simulink model "SILsim"  (R2024a)
settings: Solver=ode8  StartTime=0.0  StopTime=inf  FixedStep=SampleTime  RelTol=1e-3
values from neighbouring files (symbols this model uses):
  Arm = [ ... (first row only)    [launch.m]
  CDDrone = 0.01    [launch.m]
  CDval = 0.008    [launch.m]
  g = 9.81    [launch.m]
  m = 1    [launch.m]
  m_to_mm = 1000    [launch.m]
  prop_inertia = (1/12) * 0.015 * 0.127^2    (= 2.016125e-05)    [launch.m]
  R = 0.127    [launch.m]
  ref_height = 76    [launch.m]
  ref_lat = 437818446e-7    (= 43.7818446)    [launch.m]
  ref_lon = -794679715e-7    (= -79.4679715)    [launch.m]
  rotorRPMMax = 10000    [launch.m]
  rotorTimeConst = 0.05    [launch.m]
  SampleTime = 0.004    [launch.m]
  tilt_speed = [0; pi/4; 0]    [launch.m]
undefined symbols (not defined in the file or in its folder): contact, control, ddx, ddy, ddz, dx, dy, dz, fractalcoef, lastVh, p, pitch, q, r, roll, X, Y, yaw, Z
libraries: sharedutil x3, robotcorelib x2, simulink x2, shared6dof x1, simulink_extras x1, matrix_library x1, aerolibatmos2 x1, sensorgpslib x1, mspsensorlib x1, aerolibanimutils x1, uavutilslib x1
(part 2 of 2)

== system SILsim/Quad Tiltrotor Dynamics/Airframe/Motor Forces and Torques/If transitioning/Multirotor Subsystem/Rotor Subsystem/Force Calculation ==
  Coeff. Thrust : Inport
  Omega : Inport  Port=2
  rho : Inport  Port=3
  Tilt angle : Inport  Port=4
  Arm : Inport  Port=5
  Components : Subsystem
  Fx Sign : Subsystem
  Induced Vel Calc : Subsystem
  Math Function3 : Math  Operator=square  SignedPower=on
  Mux : Mux  Inputs=3
  Product6 : Product  Inputs=3
  R3 : Gain  Gain=R*R*pi*R*R
  Induced Velocity : Outport
  Thrust : Outport  Port=2
  wires:
  Coeff. Thrust/1 -> Product6/1
  Math Function3/1 -> R3/1
  Induced Vel Calc/1(Vh) -> Induced Velocity/1
  R3/1 -> Product6/2
  rho/1 -> Product6/3
  Omega/1 -> Math Function3/1
  Product6/1 -> Components/3(F), Induced Vel Calc/1(Thrust)  "F"
  Arm/1 -> Fx Sign/1(Arm)
  Mux/1 -> Thrust/1
  Fx Sign/1(Xsign) -> Components/1(Sign)
  Tilt angle/1 -> Components/2(Tilt angle)
  Components/1(Fx) -> Mux/1
  Components/2(Fy) -> Mux/2
  Components/3(Fz) -> Mux/3

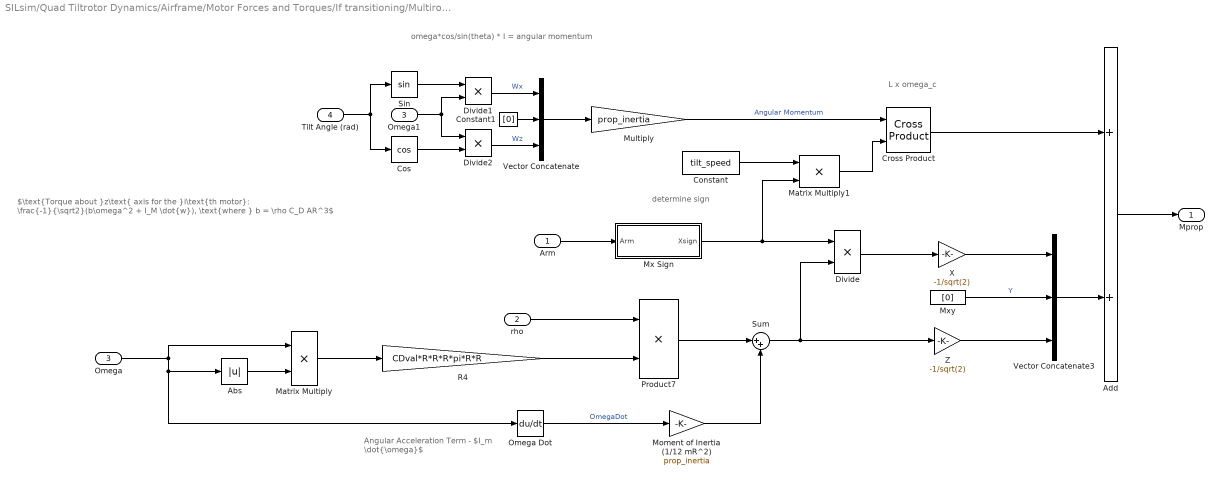
== system SILsim/Quad Tiltrotor Dynamics/Airframe/Motor Forces and Torques/If transitioning/Multirotor Subsystem/Rotor Subsystem/Moment Calculation ==
  note: determine sign
  note: L x omega_c
  note: omega*cos/sin(theta) * I = angular momentum
  note: $\text{Torque about }z\text{ axis for the }i\text{th motor}: \frac{-1}{\sqrt2}(b\omega^2 + I_M \dot{w}), \text{where } b = \rho C_D AR^3$
  note: Angular Acceleration Term - $I_m \dot{\omega}$
  Arm : Inport
  rho : Inport  Port=2
  Omega : Inport  Port=3
  Tilt Angle (rad) : Inport  Port=4
  Abs : Abs  SaturateOnIntegerOverflow=off
  Add : Sum
  Constant : Constant  Value=tilt_speed
  Constant1 : Constant  Value=[0]
  Cos : Trigonometry  Operator=cos
  Cross Product : matrix_library/Cross Product
  Divide : Product  Inputs=**
  Divide1 : Product  Inputs=**
  Divide2 : Product  Inputs=**
  Matrix Multiply : Product
  Matrix Multiply1 : Product
  Moment of Inertia (1/12 mR^2) : Gain  Gain=prop_inertia
  Multiply : Gain  Gain=prop_inertia
  Mx Sign : Subsystem
  Mxy : Constant  Value=[0]
  Omega Dot : Derivative
  Omega1 : InportShadow  Port=3
  Product7 : Product
  R4 : Gain  Gain=CDval*R*R*R*pi*R*R
  Sin : Trigonometry
  Sum : Sum  Inputs=|++
  Vector Concatenate : Concatenate  NumInputs=3
  Vector Concatenate3 : Concatenate  NumInputs=3
  X : Gain  Gain=-1/sqrt(2)
  Z : Gain  Gain=-1/sqrt(2)
  Mprop : Outport
  wires:
  R4/1 -> Product7/2
  rho/1 -> Product7/1
  Omega/1 -> Omega Dot/1, Abs/1, Matrix Multiply/1
  Omega Dot/1 -> Moment of Inertia (1/12 mR^2)/1  "OmegaDot"
  Sum/1 -> Z/1, Divide/2
  Product7/1 -> Sum/1
  Moment of Inertia (1/12 mR^2)/1 -> Sum/2
  Z/1 -> Vector Concatenate3/3
  Divide/1 -> X/1
  Mxy/1 -> Vector Concatenate3/2  "Y"
  Arm/1 -> Mx Sign/1(Arm)
  Mx Sign/1(Xsign) -> Divide/1, Matrix Multiply1/2
  Matrix Multiply/1 -> R4/1
  Abs/1 -> Matrix Multiply/2
  Tilt Angle (rad)/1 -> Cos/1, Sin/1
  Cos/1 -> Divide2/2
  Sin/1 -> Divide1/1
  Divide1/1 -> Vector Concatenate/1  "Wx"
  Vector Concatenate/1 -> Multiply/1
  Multiply/1 -> Cross Product/1  "Angular Momentum"
  Cross Product/1 -> Add/1
  Divide2/1 -> Vector Concatenate/3  "Wz"
  Constant1/1 -> Vector Concatenate/2
  Omega1/1 -> Divide2/1, Divide1/2
  Matrix Multiply1/1 -> Cross Product/2
  Constant/1 -> Matrix Multiply1/1
  X/1 -> Vector Concatenate3/1
  Vector Concatenate3/1 -> Add/2
  Add/1 -> Mprop/1

== system SILsim/Quad Tiltrotor Dynamics/Airframe/Motor Forces and Torques/If transitioning/Multirotor Subsystem/Rotor Subsystem/Tilted Ct Estimator ==
  note: - calculate ct/c0 from both estimators
      | - use tilt angle to perform a weighted average
  note: Accurate method:
      |
      | - model the tilt in ansys and find the thrust variation
  note: Possible simplified method:
      |
      | - stick to vrs dynamics from non tilted state for transitioning part -> more conservative
      | - do some interpolation between tilted and non tilted estimators
  Vz : Inport
  rpm : Inport  Port=2
  tilt_angle : Inport  Port=3
  Abs : Abs  SaturateOnIntegerOverflow=off
  Calculate Ct : Product  Inputs=**
  Ct/C0 State Switcher : Subsystem
  Ct0 estimator for RPM : Polyval  Coefs=[0.000000000012185, -0.000000274732884, 0.008305365728125]
  Divide1 : Product  Inputs=*/
  Tilt Normalization : Subsystem
  Vh Calculator : Polyval  Coefs=[-5.17622414362771e-09, 0.000822973507549008, 0.0232660553338375]
  Weighted Average Ct/C0 Fit : Subsystem
  Ct : Outport
  wires:
  Vh Calculator/1 -> Divide1/2  "Vh"
  Ct/C0 State Switcher/1(Out1) -> Calculate Ct/1  "Ct/C0"
  Divide1/1 -> Ct/C0 State Switcher/1(" Vz/Vh"), Weighted Average Ct/C0 Fit/1(Vz/Vh)  "Vz/Vh"
  rpm/1 -> Abs/1
  Abs/1 -> Vh Calculator/1, Ct0 estimator for RPM/1
  Ct0 estimator for RPM/1 -> Calculate Ct/2  "Ct0"
  Vz/1 -> Divide1/1
  Calculate Ct/1 -> Ct/1  "Ct"
  Weighted Average Ct/C0 Fit/1(Ct/Ct0) -> Ct/C0 State Switcher/2(Ct/C0 Fit)
  tilt_angle/1 -> Tilt Normalization/1(Angle)
  Tilt Normalization/1(%) -> Weighted Average Ct/C0 Fit/2(tilt %)
  Weighted Average Ct/C0 Fit/2(Ct/Ct0 Past Fit) -> Ct/C0 State Switcher/3(Ct/Ct0 Past Fit)

== system SILsim/Quad Tiltrotor Dynamics/Airframe/Motor Forces and Torques/If Tilted/Multirotor Subsystem/Rotor Subsystem/Ct Estimator/Ct//C0 State Switcher ==
  " Vz/Vh" : Inport
  Ct/C0 Fit : Inport  Port=2
  " Vz/Vh1" : InportShadow
  Constant : Constant  Value=1.00463796511
  If : If  IfExpression=u1 >= -2.828427125 & u1 <= 0  ElseIfExpressions=u1 < -2.828427125
  If Action Subsystem : Subsystem  TreatAsAtomicUnit=on
  If Action Subsystem1 : Subsystem  TreatAsAtomicUnit=on
  If Action Subsystem2 : Subsystem  TreatAsAtomicUnit=on
  Merge : Merge  Inputs=3
  Scope1 : Scope
  Out1 : Outport
  wires:
  If Action Subsystem2/1(Out1) -> Merge/3
  If/3 -> If Action Subsystem2/Action  "climb"
  If/1 -> If Action Subsystem/Action  "descent"
  If Action Subsystem/1(Out1) -> Merge/1
  " Vz/Vh"/1 -> If/1
  If/2 -> If Action Subsystem1/Action  "past curve fit"
  Merge/1 -> Scope1/1, Out1/1
  Ct/C0 Fit/1 -> If Action Subsystem/1(In1)
  Constant/1 -> If Action Subsystem2/1("  ")
  If Action Subsystem1/1(" ") -> Merge/2
  " Vz/Vh1"/1 -> If Action Subsystem1/1(" Vz/Vh")

== system SILsim/Quad Tiltrotor Dynamics/Airframe/Motor Forces and Torques/If Tilted/Multirotor Subsystem/Rotor Subsystem/Force Calculation/Fx Sign ==
  Arm : Inport
  Sign : Signum
  X selector : Selector  InputPortWidth=3  IndexOptions=Index vector (dialog)  Indices=[1]  OutputSizes=1
  Xsign : Outport
  wires:
  Arm/1 -> X selector/1
  X selector/1 -> Sign/1
  Sign/1 -> Xsign/1

== system SILsim/Quad Tiltrotor Dynamics/Airframe/Motor Forces and Torques/If Tilted/Multirotor Subsystem/Rotor Subsystem/Force Calculation/Induced Vel Calc ==
  Thrust : Inport
  Denom : Constant  Value=2*1.225*pi*R^2
  Divide : Product  Inputs=*/
  Sqrt : Sqrt  OutDataTypeStr=double
  Vh : Outport
  wires:
  Denom/1 -> Divide/2
  Divide/1 -> Sqrt/1
  Sqrt/1 -> Vh/1
  Thrust/1 -> Divide/1

== system SILsim/Quad Tiltrotor Dynamics/Airframe/Motor Forces and Torques/If Tilted/Multirotor Subsystem/Rotor Subsystem/Moment Calculation/Mx Sign ==
  Arm : Inport
  Sign : Signum
  X selector : Selector  InputPortWidth=3  IndexOptions=Index vector (dialog)  Indices=[1]  OutputSizes=1
  Xsign : Outport
  wires:
  Arm/1 -> X selector/1
  X selector/1 -> Sign/1
  Sign/1 -> Xsign/1

== system SILsim/Quad Tiltrotor Dynamics/Airframe/Motor Forces and Torques/If non tilted/Multirotor Subsystem/Rotor Subsystem/Force Calculation/Induced Vel Calc ==
  Thrust : Inport
  Denom : Constant  Value=2*1.225*pi*R^2
  Divide : Product  Inputs=*/
  Saturation : Saturate  UpperLimit=inf  LowerLimit=0
  Sqrt : Sqrt  OutDataTypeStr=double
  Vh : Outport
  wires:
  Denom/1 -> Divide/2
  Divide/1 -> Saturation/1
  Sqrt/1 -> Vh/1
  Thrust/1 -> Divide/1
  Saturation/1 -> Sqrt/1

== system SILsim/Quad Tiltrotor Dynamics/Airframe/Motor Forces and Torques/If non tilted/Multirotor Subsystem/Rotor Subsystem/Non Tilted Ct estimator/Ct//C0 State Switcher ==
  note: add random number variations to VRS thrust to simulate thrust fluctuations
  " Vz/Vh" : Inport
  Ct/C0 Fit : Inport  Port=2
  " Vz/Vh1" : InportShadow
  Climb : Subsystem  TreatAsAtomicUnit=on
  Constant : Constant  Value=0.9905
  Descent : Subsystem  TreatAsAtomicUnit=on
  If : If  IfExpression=u1 >= -2 & u1 <= 0  ElseIfExpressions=u1 < -2
  Merge : Merge  Inputs=3
  Past Curve Fit : Subsystem  TreatAsAtomicUnit=on
  Ct/Ct0 : Outport
  wires:
  Past Curve Fit/1(" ") -> Merge/2
  Climb/1(Out1) -> Merge/3
  If/3 -> Climb/Action
  If/1 -> Descent/Action
  If/2 -> Past Curve Fit/Action
  Ct/C0 Fit/1 -> Descent/1(Ct_Ct0)
  " Vz/Vh1"/1 -> Past Curve Fit/1(" Vz/Vh")
  Constant/1 -> Climb/1("  ")
  Merge/1 -> Ct/Ct0/1
  " Vz/Vh"/1 -> If/1
  Descent/1(Outport) -> Merge/1

== system SILsim/Quad Tiltrotor Dynamics/Airframe/Motor Forces and Torques/If transitioning/Multirotor Subsystem/Rotor Subsystem/Force Calculation/Components ==
  Sign : Inport
  Tilt angle : Inport  Port=2
  F : Inport  Port=3
  Constant : Constant  Value=0
  Cos : Trigonometry
  Divide : Product  Inputs=**
  Matrix Multiply : Product
  Matrix Multiply1 : Product
  Sin : Trigonometry  Operator=cos
  Fx : Outport
  Fy : Outport  Port=2
  Fz : Outport  Port=3
  wires:
  Tilt angle/1 -> Cos/1, Sin/1
  Sign/1 -> Divide/1
  Sin/1 -> Matrix Multiply1/1
  Constant/1 -> Fy/1  "Fy"
  Cos/1 -> Matrix Multiply/2
  Matrix Multiply/1 -> Fx/1  "Fx"
  Divide/1 -> Matrix Multiply/1
  F/1 -> Matrix Multiply1/2, Divide/2
  Matrix Multiply1/1 -> Fz/1  "Fz"

== system SILsim/Quad Tiltrotor Dynamics/Airframe/Motor Forces and Torques/If transitioning/Multirotor Subsystem/Rotor Subsystem/Force Calculation/Fx Sign ==
  Arm : Inport
  Sign : Signum
  X selector : Selector  InputPortWidth=3  IndexOptions=Index vector (dialog)  Indices=[1]  OutputSizes=1
  Xsign : Outport
  wires:
  Arm/1 -> X selector/1
  X selector/1 -> Sign/1
  Sign/1 -> Xsign/1

== system SILsim/Quad Tiltrotor Dynamics/Airframe/Motor Forces and Torques/If transitioning/Multirotor Subsystem/Rotor Subsystem/Force Calculation/Induced Vel Calc ==
  Thrust : Inport
  Denom : Constant  Value=2*1.225*pi*R^2
  Divide : Product  Inputs=*/
  Sqrt : Sqrt  OutDataTypeStr=double
  Vh : Outport
  wires:
  Denom/1 -> Divide/2
  Divide/1 -> Sqrt/1
  Sqrt/1 -> Vh/1
  Thrust/1 -> Divide/1

== system SILsim/Quad Tiltrotor Dynamics/Airframe/Motor Forces and Torques/If transitioning/Multirotor Subsystem/Rotor Subsystem/Moment Calculation/Mx Sign ==
  Arm : Inport
  Sign : Signum
  X selector : Selector  InputPortWidth=3  IndexOptions=Index vector (dialog)  Indices=[1]  OutputSizes=1
  Xsign : Outport
  wires:
  Arm/1 -> X selector/1
  X selector/1 -> Sign/1
  Sign/1 -> Xsign/1

== system SILsim/Quad Tiltrotor Dynamics/Airframe/Motor Forces and Torques/If transitioning/Multirotor Subsystem/Rotor Subsystem/Tilted Ct Estimator/Ct//C0 State Switcher ==
  " Vz/Vh" : Inport
  Ct/C0 Fit : Inport  Port=2
  Ct/Ct0 Past Fit : Inport  Port=3
  Constant : Constant  Value=1.00463796511
  If : If  IfExpression=u1 >= -2 & u1 <= 0  ElseIfExpressions=u1 < -2
  If Action Subsystem : Subsystem  TreatAsAtomicUnit=on
  If Action Subsystem1 : Subsystem  TreatAsAtomicUnit=on
  If Action Subsystem2 : Subsystem  TreatAsAtomicUnit=on
  Merge : Merge  Inputs=3
  Out1 : Outport
  wires:
  If Action Subsystem1/1(" ") -> Merge/2
  If Action Subsystem2/1(Out1) -> Merge/3
  If/3 -> If Action Subsystem2/Action  "climb"
  If/1 -> If Action Subsystem/Action  "descent"
  If Action Subsystem/1(Out1) -> Merge/1
  " Vz/Vh"/1 -> If/1
  If/2 -> If Action Subsystem1/Action  "past curve fit"
  Merge/1 -> Out1/1
  Ct/C0 Fit/1 -> If Action Subsystem/1(In1)
  Constant/1 -> If Action Subsystem2/1("  ")
  Ct/Ct0 Past Fit/1 -> If Action Subsystem1/1(Inport)

== system SILsim/Quad Tiltrotor Dynamics/Airframe/Motor Forces and Torques/If transitioning/Multirotor Subsystem/Rotor Subsystem/Tilted Ct Estimator/Tilt Normalization ==
  Angle : Inport
  Constant1 : Constant  Value=pi/4
  Divide2 : Product  Inputs=*/
  % : Outport
  wires:
  Constant1/1 -> Divide2/2
  Divide2/1 -> %/1
  Angle/1 -> Divide2/1

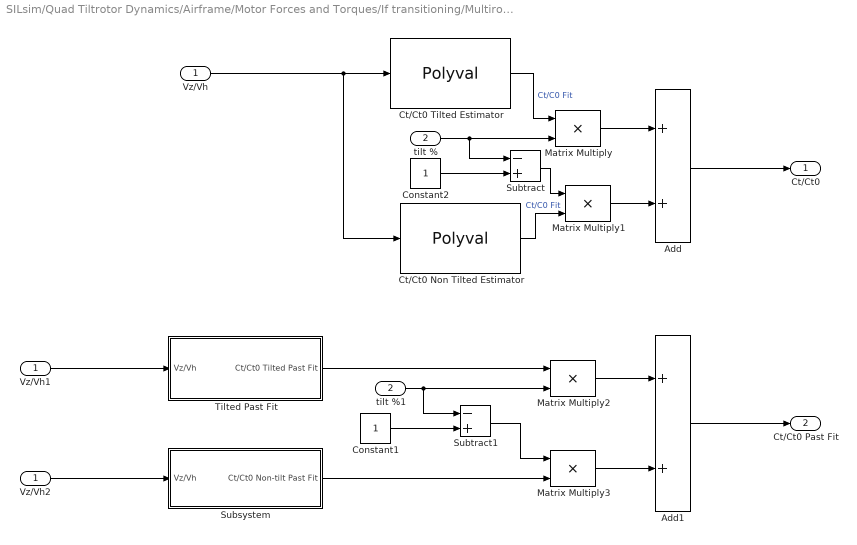
== system SILsim/Quad Tiltrotor Dynamics/Airframe/Motor Forces and Torques/If transitioning/Multirotor Subsystem/Rotor Subsystem/Tilted Ct Estimator/Weighted Average Ct//C0 Fit ==
  Vz/Vh : Inport
  tilt % : Inport  Port=2
  Add : Sum
  Add1 : Sum
  Constant1 : Constant
  Constant2 : Constant
  Ct/Ct0 Non Tilted Estimator : Polyval  Coefs=[0.147117704259973, 0.135195473604728, -0.341999514591595, -0.246799876690693, 0.999678014049876]
  Ct/Ct0 Tilted Estimator : Polyval  Coefs=[-0.012716815691322, -0.022830541813396, 0.156313447084851, -0.031641009616291, 1.004637965110952]
  Matrix Multiply{,1..3} (4 alike) : Product
  Subsystem : Subsystem
  Subtract : Sum  Inputs=-+
  Subtract1 : Sum  Inputs=-+
  Tilted Past Fit : Subsystem
  Vz/Vh1 : InportShadow
  Vz/Vh2 : InportShadow
  tilt %1 : InportShadow  Port=2
  Ct/Ct0 : Outport
  Ct/Ct0 Past Fit : Outport  Port=2
  wires:
  Ct/Ct0 Tilted Estimator/1 -> Matrix Multiply/1  "Ct/C0 Fit"
  Vz/Vh/1 -> Ct/Ct0 Non Tilted Estimator/1, Ct/Ct0 Tilted Estimator/1
  Matrix Multiply/1 -> Add/1
  Ct/Ct0 Non Tilted Estimator/1 -> Matrix Multiply1/2  "Ct/C0 Fit"
  Matrix Multiply1/1 -> Add/2
  Subtract/1 -> Matrix Multiply1/1
  Add/1 -> Ct/Ct0/1
  Vz/Vh1/1 -> Tilted Past Fit/1(Vz/Vh)
  Vz/Vh2/1 -> Subsystem/1(" Vz/Vh")
  Add1/1 -> Ct/Ct0 Past Fit/1
  Constant2/1 -> Subtract/2
  tilt %/1 -> Subtract/1, Matrix Multiply/2
  Constant1/1 -> Subtract1/2
  Matrix Multiply2/1 -> Add1/1
  Matrix Multiply3/1 -> Add1/2
  tilt %1/1 -> Subtract1/1, Matrix Multiply2/2
  Subtract1/1 -> Matrix Multiply3/1
  Tilted Past Fit/1(Ct/Ct0 Tilted Past Fit) -> Matrix Multiply2/1
  Subsystem/1(Ct/Ct0 Non-tilt Past Fit) -> Matrix Multiply3/2

== system SILsim/Quad Tiltrotor Dynamics/Airframe/Motor Forces and Torques/If Tilted/Multirotor Subsystem/Rotor Subsystem/Ct Estimator/Ct//C0 State Switcher/If Action Subsystem ==
  In1 : Inport
  Action Port : ActionPort  ActionPortLabel=if(u1 >= -2.828427125 & u1 <= 0)
  Out1 : Outport
  wires:
  In1/1 -> Out1/1

== system SILsim/Quad Tiltrotor Dynamics/Airframe/Motor Forces and Torques/If Tilted/Multirotor Subsystem/Rotor Subsystem/Ct Estimator/Ct//C0 State Switcher/If Action Subsystem1 ==
  note: 1/2 * ln(-(x+1.23626605195)) + 1.814813688
  " Vz/Vh" : Inport
  Action Port : ActionPort  ActionPortLabel=elseif(u1 < -2.828427125)
  Add : Sum
  Constant : Constant  Value=1.814813688
  Constant1 : Constant  Value=1.23626605195
  Gain : Gain  Gain=1/2
  Multiply : Gain  Gain=-1
  Saturation : Saturate  UpperLimit=inf  LowerLimit=0.001
  Sum : Sum  Inputs=|++
  ln : Math  Operator=log
  " " : Outport
  wires:
  Gain/1 -> Add/1
  Constant/1 -> Add/2
  " Vz/Vh"/1 -> Sum/1
  Sum/1 -> Multiply/1
  Constant1/1 -> Sum/2
  Add/1 -> " "/1
  Multiply/1 -> Saturation/1
  ln/1 -> Gain/1
  Saturation/1 -> ln/1

== system SILsim/Quad Tiltrotor Dynamics/Airframe/Motor Forces and Torques/If Tilted/Multirotor Subsystem/Rotor Subsystem/Ct Estimator/Ct//C0 State Switcher/If Action Subsystem2 ==
  "  " : Inport
  Action Port : ActionPort  ActionPortLabel=else
  Out1 : Outport
  wires:
  "  "/1 -> Out1/1

== system SILsim/Quad Tiltrotor Dynamics/Airframe/Motor Forces and Torques/If non tilted/Multirotor Subsystem/Rotor Subsystem/Non Tilted Ct estimator/Ct//C0 State Switcher/Climb ==
  "  " : Inport
  Action Port : ActionPort  ActionPortLabel=else
  Out1 : Outport
  wires:
  "  "/1 -> Out1/1

== system SILsim/Quad Tiltrotor Dynamics/Airframe/Motor Forces and Torques/If non tilted/Multirotor Subsystem/Rotor Subsystem/Non Tilted Ct estimator/Ct//C0 State Switcher/Descent ==
  Ct_Ct0 : Inport
  Action Port : ActionPort  ActionPortLabel=if(u1 >= -2 & u1 <= 0)
  Outport : Outport
  wires:
  Ct_Ct0/1 -> Outport/1

== system SILsim/Quad Tiltrotor Dynamics/Airframe/Motor Forces and Torques/If non tilted/Multirotor Subsystem/Rotor Subsystem/Non Tilted Ct estimator/Ct//C0 State Switcher/Past Curve Fit ==
  note: 1/2*ln(-(x+1.7439783573836165)) + 2.07884583669
  " Vz/Vh" : Inport
  Action Port : ActionPort  ActionPortLabel=elseif(u1 < -2)
  Add : Sum
  Constant : Constant  Value=2.07884583669
  Constant1 : Constant  Value=1.7439783573836165
  Gain : Gain  Gain=1/2
  Multiply : Gain  Gain=-1
  Saturation : Saturate  UpperLimit=inf  LowerLimit=0.0001
  Sum : Sum  Inputs=|++
  ln : Math  Operator=log
  " " : Outport
  wires:
  Add/1 -> " "/1
  Constant/1 -> Add/2
  Multiply/1 -> Saturation/1
  ln/1 -> Gain/1
  " Vz/Vh"/1 -> Sum/1
  Sum/1 -> Multiply/1
  Constant1/1 -> Sum/2
  Gain/1 -> Add/1
  Saturation/1 -> ln/1

== system SILsim/Quad Tiltrotor Dynamics/Airframe/Motor Forces and Torques/If transitioning/Multirotor Subsystem/Rotor Subsystem/Tilted Ct Estimator/Ct//C0 State Switcher/If Action Subsystem ==
  In1 : Inport
  Action Port : ActionPort  ActionPortLabel=if(u1 >= -2 & u1 <= 0)
  Out1 : Outport
  wires:
  In1/1 -> Out1/1

== system SILsim/Quad Tiltrotor Dynamics/Airframe/Motor Forces and Torques/If transitioning/Multirotor Subsystem/Rotor Subsystem/Tilted Ct Estimator/Ct//C0 State Switcher/If Action Subsystem1 ==
  Inport : Inport
  Action Port : ActionPort  ActionPortLabel=elseif(u1 < -2)
  " " : Outport
  wires:
  Inport/1 -> " "/1

== system SILsim/Quad Tiltrotor Dynamics/Airframe/Motor Forces and Torques/If transitioning/Multirotor Subsystem/Rotor Subsystem/Tilted Ct Estimator/Ct//C0 State Switcher/If Action Subsystem2 ==
  "  " : Inport
  Action Port : ActionPort  ActionPortLabel=else
  Out1 : Outport
  wires:
  "  "/1 -> Out1/1

== system SILsim/Quad Tiltrotor Dynamics/Airframe/Motor Forces and Torques/If transitioning/Multirotor Subsystem/Rotor Subsystem/Tilted Ct Estimator/Weighted Average Ct//C0 Fit/Subsystem ==
  " Vz/Vh" : Inport
  Add2 : Sum
  Constant : Constant  Value=2.07884583669
  Constant3 : Constant  Value=1.7439783573836165
  Gain : Gain  Gain=1/2
  Multiply : Gain  Gain=-1
  Saturation : Saturate  UpperLimit=inf  LowerLimit=0.0001
  Sum : Sum  Inputs=|++
  ln : Math  Operator=log
  Ct/Ct0 Non-tilt Past Fit : Outport
  wires:
  ln/1 -> Gain/1
  Sum/1 -> Multiply/1
  " Vz/Vh"/1 -> Sum/1
  Add2/1 -> Ct/Ct0 Non-tilt Past Fit/1
  Saturation/1 -> ln/1
  Multiply/1 -> Saturation/1
  Constant3/1 -> Sum/2
  Gain/1 -> Add2/1
  Constant/1 -> Add2/2

== system SILsim/Quad Tiltrotor Dynamics/Airframe/Motor Forces and Torques/If transitioning/Multirotor Subsystem/Rotor Subsystem/Tilted Ct Estimator/Weighted Average Ct//C0 Fit/Tilted Past Fit ==
  Vz/Vh : Inport
  Add1 : Sum
  Constant : Constant  Value=1.814813688
  Constant3 : Constant  Value=1.23626605195
  Gain : Gain  Gain=1/2
  Multiply : Gain  Gain=-1
  Saturation : Saturate  UpperLimit=inf  LowerLimit=0.001
  Sum : Sum  Inputs=|++
  ln : Math  Operator=log
  Ct/Ct0 Tilted Past Fit : Outport
  wires:
  Gain/1 -> Add1/1
  Saturation/1 -> ln/1
  Constant3/1 -> Sum/2
  Vz/Vh/1 -> Sum/1
  ln/1 -> Gain/1
  Multiply/1 -> Saturation/1
  Constant/1 -> Add1/2
  Add1/1 -> Ct/Ct0 Tilted Past Fit/1
  Sum/1 -> Multiply/1

== matlab function SILsim/Quad Tiltrotor Dynamics/Airframe/Motor Forces and Torques/If transitioning/Multirotor Subsystem/Rotor Subsystem/Induced Vel Convergence Checker ==
  data: rpmToCalc output; newVh output; Converged output; Vh input; convergence_threshold parameter; lastVh input
function [rpmToCalc, newVh, Converged] = CalculateInducedVelocity(Vh, convergence_threshold, lastVh)

    % Initialize variables
    persistent rpm_index rpm_values Vh_values exportedCoefficients;

    if isempty(rpm_index)
        rpm_index = 1;
        rpm_values = 1:1000:10001;
        Vh_values = zeros(size(rpm_values));
        exportedCoefficients = false;
    end

    if rpm_index > 11
        rpmToCalc = 1;
        newVh = 0.1;
        Converged = 1;
        return;
    end

    % Calculate the difference between the current and last induced velocity
    difference = abs(Vh - lastVh);
    rpmToCalc = rpm_values(rpm_index);

    if difference < convergence_threshold
        % Convergence achieved
        Converged = 1;
        newVh = Vh; % Update to the current induced velocity
        Vh_values(rpm_index) = Vh;
        
        if rpm_index >= length(rpm_values) && exportedCoefficients == false
            coefficients = fitVhToRPM(rpm_values, Vh_values);
            assignin('base', 'coefficients', coefficients);
            assignin('base', 'rpm_values', rpm_values);
            assignin('base', 'Vh_values', Vh_values);
            exportedCoefficients = true;
            return;
        else
            if rpm_index ~= 11
                rpmToCalc = rpm_values(rpm_index+1);
            end
        end

        % Move to the next RPM value
        if rpm_index < 11
            rpm_index = rpm_index + 1;
        end
    else
        % Convergence not achieved
        Converged = 0;
        newVh = Vh; % Update to the new induced velocity
    end
end

function coefficients = fitVhToRPM(rpm_values, Vh_values)
    % Fit a polynomial (or any other function) to the RPM and Vh values
    p = polyfit(rpm_values, Vh_values, 2);
    coefficients = p;
end

== matlab function SILsim/Quad Tiltrotor Dynamics/Airframe/Motor Forces and Torques/If non tilted/Multirotor Subsystem/Rotor Subsystem/Induced Vel Convergence Checker ==
  data: rpmToCalc output; newVh output; Converged output; Vh input; convergence_threshold parameter; lastVh input
function [rpmToCalc, newVh, Converged] = CalculateInducedVelocity(Vh, convergence_threshold, lastVh)

    % Initialize variables
    persistent rpm_index rpm_values Vh_values exportedCoefficients;

    if isempty(rpm_index)
        rpm_index = 1;
        rpm_values = 1:1000:10001;
        Vh_values = zeros(size(rpm_values));
        exportedCoefficients = false;
    end

    if rpm_index > 11
        rpmToCalc = 1;
        newVh = 0.1;
        Converged = 1;
        return;
    end

    % Calculate the difference between the current and last induced velocity
    difference = abs(Vh - lastVh);
    rpmToCalc = rpm_values(rpm_index);

    if difference < convergence_threshold
        % Convergence achieved
        Converged = 1;
        newVh = Vh; % Update to the current induced velocity
        Vh_values(rpm_index) = Vh;
        
        if rpm_index >= length(rpm_values) && exportedCoefficients == false
            coefficients = fitVhToRPM(rpm_values, Vh_values);
            assignin('base', 'coefficients', coefficients);
            assignin('base', 'rpm_values', rpm_values);
            assignin('base', 'Vh_values', Vh_values);
            exportedCoefficients = true;
            return;
        else
            if rpm_index ~= 11
                rpmToCalc = rpm_values(rpm_index+1);
            end
        end

        % Move to the next RPM value
        if rpm_index < 11
            rpm_index = rpm_index + 1;
        end
    else
        % Convergence not achieved
        Converged = 0;
        newVh = Vh; % Update to the new induced velocity
    end
end

function coefficients = fitVhToRPM(rpm_values, Vh_values)
    % Fit a polynomial (or any other function) to the RPM and Vh values
    p = polyfit(rpm_values, Vh_values, 2);
    coefficients = p;
end

== matlab function SILsim/Quad Tiltrotor Dynamics/Airframe/Motor Forces and Torques/If Tilted/Multirotor Subsystem/Rotor Subsystem/Induced Vel Convergence Checker ==
  data: rpmToCalc output; newVh output; Converged output; Vh input; convergence_threshold parameter; lastVh input
function [rpmToCalc, newVh, Converged] = CalculateInducedVelocity(Vh, convergence_threshold, lastVh)

    % Initialize variables
    persistent rpm_index rpm_values Vh_values exportedCoefficients;

    if isempty(rpm_index)
        rpm_index = 1;
        rpm_values = 1:1000:10001;
        Vh_values = zeros(size(rpm_values));
        exportedCoefficients = false;
    end

    if rpm_index > 11
        rpmToCalc = 1;
        newVh = 0.1;
        Converged = 1;
        return;
    end

    % Calculate the difference between the current and last induced velocity
    difference = abs(Vh - lastVh);
    rpmToCalc = rpm_values(rpm_index);

    if difference < convergence_threshold
        % Convergence achieved
        Converged = 1;
        newVh = Vh; % Update to the current induced velocity
        Vh_values(rpm_index) = Vh;
        
        if rpm_index >= length(rpm_values) && exportedCoefficients == false
            coefficients = fitVhToRPM(rpm_values, Vh_values);
            assignin('base', 'coefficients', coefficients);
            assignin('base', 'rpm_values', rpm_values);
            assignin('base', 'Vh_values', Vh_values);
            exportedCoefficients = true;
            return;
        else
            if rpm_index ~= 11
                rpmToCalc = rpm_values(rpm_index+1);
            end
        end

        % Move to the next RPM value
        if rpm_index < 11
            rpm_index = rpm_index + 1;
        end
    else
        % Convergence not achieved
        Converged = 0;
        newVh = Vh; % Update to the new induced velocity
    end
end

function coefficients = fitVhToRPM(rpm_values, Vh_values)
    % Fit a polynomial (or any other function) to the RPM and Vh values
    p = polyfit(rpm_values, Vh_values, 2);
    coefficients = p;
end
